simulink model "xPC_parker"  (Simulink 8.5)
settings: Solver=FixedStepDiscrete  StartTime=0.0  StopTime=inf  FixedStep=dts  RelTol=1e-3
InitFcn:
  | PARKER_DEPENDENCY
  | Parker_Multi_Axis_Init
  | Parker_ATI_Init
  | Parker_Home_Init
  | Parker_Davinci_Init
  | Parker_UDP_Init
  | Parker_LinIntPathPlan_Init
  | Parker_ScopeFormat_Init
  | Parker_magnetic_init
undefined symbols (not defined in the file): A, accel_filter_coeffs, ATI_torque_Nmm, B, counter_offset, DavinciFilterDen, DavinciFilterNum, DesiredPath, dt, dt_ENC, dt_trakstar, dts, dtudp, ENC_obs_filter_coeffs, encoder_counts, F, f_mag_desired_shape, filter_coeffs_bias, force_bias, forceDeadZone, FT_unbias_time, grav_vector, Home_in_TKbase, HOMING_dx, HOMING_num_joint, HOMING_tspan, HOMING_Vmov, inv_T, JOINT_Limits_Negative, JOINT_Limits_Postive, Kd, Ki_force, Kp, Kp_force, Kv_force, Low, N_acceleration, N_bias, N_ENC_obs_filter, N_obs_velocity, N_trakstar, N_velocity, Omega7IsLeftHanded, omni_scaling, PathPlanSpeed, pitch, quadrature_mode, R_FT2robot, R_omni, R_robot2TKbase, ResRateEpsilon, ResRateVelLimits, ResRateVelRatios, SafetyMargin, screw_pitch, torque_constant, trakstar_filter_coeffs, UDP_EN_Data2CMU, UDP_EN_DynAna, UDP_EN_VFRec ... (+6)
libraries: slrtlib x25, simulink x24, dspswit3 x15, xpcobsoletelib x15, xpcrtudplib x14, powerlib_meascontrol x3, xpcmeasurementcomputinglib x3, xpcconteclib x3
(part 3 of 3)

== system xPC_parker/Trajectory Planner/Task Input/UDP Visualize Superim ==
  x_ctr : Inport
  superim_cmd : Inport  Port=2
  Enable : EnablePort
  Demux1 : Demux  Outputs=7
  Mux3 : Mux  Inputs=3
  Pack : xpcobsoletelib/Utilities/Pack   datatypes={'double' 'double' 'double' 'double' 'double' 'double' 'double'}  byteAlign=1
  Parker_Send_to_VisualSuperim : xpcrtudplib/Legacy UDP/Send   ipAddress=255.255.255.255  ipPort=UDP_PORT_Send2VisualSuperim  localPort=-1  vblLen=off  sampletime=dtUDP_Data
  Rate Transition2 : RateTransition  OutPortSampleTime=dtUDP_Data
  STOP : Constant  Value=UDP_STOP
  wires:
  Pack/1 -> Parker_Send_to_VisualSuperim/1
  Mux3/1 -> Rate Transition2/1
  Rate Transition2/1 -> Demux1/1
  STOP/1 -> Mux3/3
  x_ctr/1 -> Mux3/1
  superim_cmd/1 -> Mux3/2
  Demux1/7 -> Pack/7
  Demux1/5 -> Pack/5
  Demux1/6 -> Pack/6
  Demux1/4 -> Pack/4
  Demux1/2 -> Pack/2
  Demux1/1 -> Pack/1
  Demux1/3 -> Pack/3

== system xPC_parker/Trajectory Planner/Task Input/position velocity acceleration ==
  velocity : Inport
  position : Inport  Port=2
  Desired Position : Subsystem
  Discrete Derivative1 : simulink/Discrete/Discrete Derivative  gainval=1.0  ICPrevScaledInput=[0;0;0]  InputProcessing=Inherited  OutMin=[]  OutMax=[]  OutDataType=fixdt(1, 16)  OutScaling=2^-10  DoSatur=off
  Mux : Mux  Inputs=3
  SatAcc : Saturate  UpperLimit=30  LowerLimit=-30
  PVA : Outport
  wires:
  Discrete Derivative1/1 -> SatAcc/1
  Mux/1 -> PVA/1
  SatAcc/1 -> Mux/3
  velocity/1 -> Desired Position/2(vel), Discrete Derivative1/1, Mux/2  "velocity"
  position/1 -> Desired Position/1(Pc)
  Desired Position/1(p_cmd) -> Mux/1

== system xPC_parker/Hybrid Motion PD Inverse Dynamics/Surf Norm Command/Conflict Check/Angle Compensation ==
  default_n : Inport
  surf_norm : Inport  Port=2
  Compensation : MATLAB Function  TreatAsAtomicUnit=on
  Constant : Constant  Value=12*pi/180
  Out1 : Outport
  wires:
  default_n/1 -> Compensation/2(N)
  surf_norm/1 -> Compensation/1(F)
  Constant/1 -> Compensation/3(angle_limit)
  Compensation/1(y) -> Out1/1

== system xPC_parker/Parker 404XR/Magnetic Tracker 125 Hz/process trak1/Filter1 ==
  in : Inport
  Discrete FIR Filter : DiscreteFir  CoefSource=Input port  SampleTime=dt_trakstar  AccumDataTypeStr=Inherit: Same as product output
  Gain : Gain  Gain=1/N_trakstar  SampleTime=dt_trakstar
  trakstar_filter_coeffs : Constant  Value=trakstar_filter_coeffs  SampleTime=dt_trakstar
  out : Outport
  wires:
  Gain/1 -> out/1
  in/1 -> Discrete FIR Filter/1
  Discrete FIR Filter/1 -> Gain/1
  trakstar_filter_coeffs/1 -> Discrete FIR Filter/2

== system xPC_parker/Parker 404XR/Magnetic Tracker 125 Hz/process trak2/Filter1 ==
  in : Inport
  Discrete FIR Filter : DiscreteFir  CoefSource=Input port  SampleTime=dt_trakstar  AccumDataTypeStr=Inherit: Same as product output
  Gain : Gain  Gain=1/N_trakstar  SampleTime=dt_trakstar
  trakstar_filter_coeffs : Constant  Value=trakstar_filter_coeffs  SampleTime=dt_trakstar
  out : Outport
  wires:
  trakstar_filter_coeffs/1 -> Discrete FIR Filter/2
  Discrete FIR Filter/1 -> Gain/1
  in/1 -> Discrete FIR Filter/1
  Gain/1 -> out/1

== system xPC_parker/Parker 404XR/Magnetic Tracker 125 Hz/process trak3/Filter1 ==
  in : Inport
  Discrete FIR Filter : DiscreteFir  CoefSource=Input port  SampleTime=dt_trakstar  AccumDataTypeStr=Inherit: Same as product output
  Gain : Gain  Gain=1/N_trakstar  SampleTime=dt_trakstar
  trakstar_filter_coeffs : Constant  Value=trakstar_filter_coeffs  SampleTime=dt_trakstar
  out : Outport
  wires:
  Gain/1 -> out/1
  in/1 -> Discrete FIR Filter/1
  Discrete FIR Filter/1 -> Gain/1
  trakstar_filter_coeffs/1 -> Discrete FIR Filter/2

== system xPC_parker/Parker 404XR/Magnetic Tracker 125 Hz/process trak4/Filter1 ==
  in : Inport
  Discrete FIR Filter : DiscreteFir  CoefSource=Input port  SampleTime=dt_trakstar  AccumDataTypeStr=Inherit: Same as product output
  Gain : Gain  Gain=1/N_trakstar  SampleTime=dt_trakstar
  trakstar_filter_coeffs : Constant  Value=trakstar_filter_coeffs  SampleTime=dt_trakstar
  out : Outport
  wires:
  trakstar_filter_coeffs/1 -> Discrete FIR Filter/2
  Discrete FIR Filter/1 -> Gain/1
  in/1 -> Discrete FIR Filter/1
  Gain/1 -> out/1

== system xPC_parker/Trajectory Planner/DaVinci MTM port: 2/DaVinci MTM/MTM Filter ==
  current_position : Inport
  Discrete FIR Filter : DiscreteFir  CoefSource=Input port  AccumDataTypeStr=Inherit: Same as product output
  Gain : Gain  Gain=1/20
  vel_filter_coeffs : Constant  Value=ones(20,1)
  vel_out : Outport
  wires:
  current_position/1 -> Discrete FIR Filter/1
  Gain/1 -> vel_out/1
  vel_filter_coeffs/1 -> Discrete FIR Filter/2
  Discrete FIR Filter/1 -> Gain/1

== system xPC_parker/Trajectory Planner/DaVinci MTM port: 2/UDP_feedback_to_MTM/Force Filter for MTM ==
  V_in : Inport  SampleTime=dts
  Discrete FIR Filter : DiscreteFir  CoefSource=Input port  SampleTime=dts  AccumDataTypeStr=Inherit: Same as product output
  Gain : Gain  Gain=1/100  SampleTime=dts
  filter_coeffs : Constant  Value=ones(100,1)  SampleTime=dt
  V_Out : Outport  SampleTime=dts
  wires:
  Gain/1 -> V_Out/1
  filter_coeffs/1 -> Discrete FIR Filter/2
  Discrete FIR Filter/1 -> Gain/1
  V_in/1 -> Discrete FIR Filter/1

== system xPC_parker/Trajectory Planner/Omega7/Feedback_to_omega7/force feedback filter ==
  V_in : Inport  SampleTime=dts
  Discrete FIR Filter : DiscreteFir  CoefSource=Input port  SampleTime=dts  AccumDataTypeStr=Inherit: Same as product output
  Gain : Gain  Gain=1/20  SampleTime=dts
  force feedback filter coef : Constant  Value=ones(20,1)  SampleTime=dts
  V_Out : Outport  SampleTime=dts
  wires:
  V_in/1 -> Discrete FIR Filter/1
  Discrete FIR Filter/1 -> Gain/1
  force feedback filter coef/1 -> Discrete FIR Filter/2
  Gain/1 -> V_Out/1

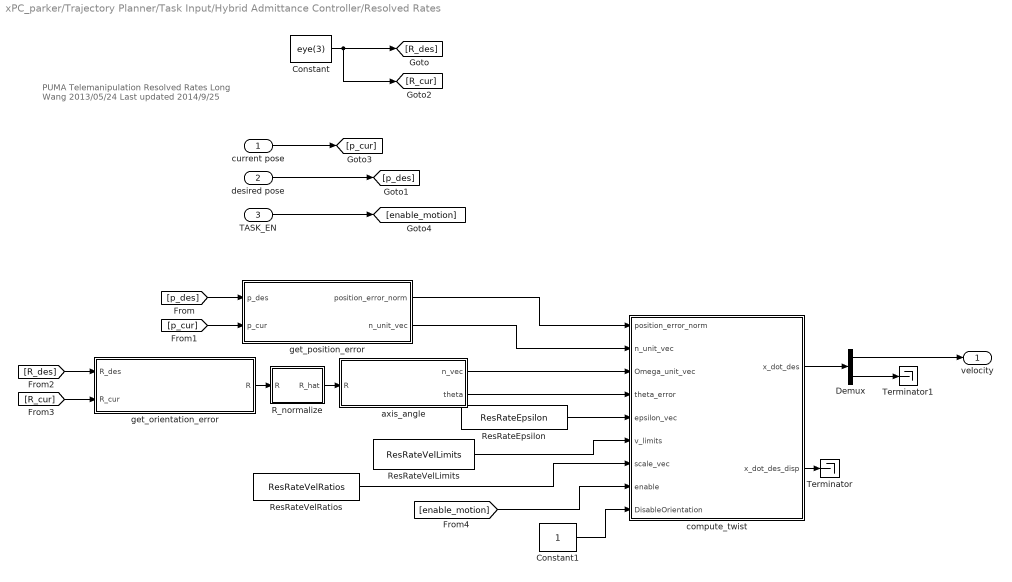
== system xPC_parker/Trajectory Planner/Task Input/Hybrid Admittance Controller/Resolved Rates ==
  note: PUMA Telemanipulation Resolved Rates
      | Long Wang
      | 2013/05/24
      | Last updated 2014/9/25
  current pose : Inport
  desired pose : Inport  Port=2
  TASK_EN : Inport  Port=3
  Constant : Constant  Value=eye(3)
  Constant1 : Constant
  Demux : Demux  Outputs=2
  R_normalize : MATLAB Function  TreatAsAtomicUnit=on
  ResRateEpsilon : Constant  Value=ResRateEpsilon
  ResRateVelLimits : Constant  Value=ResRateVelLimits
  ResRateVelRatios : Constant  Value=ResRateVelRatios
  Terminator : Terminator
  Terminator1 : Terminator
  axis_angle : MATLAB Function  TreatAsAtomicUnit=on
  compute_twist : MATLAB Function  TreatAsAtomicUnit=on
  get_orientation_error : MATLAB Function  TreatAsAtomicUnit=on
  get_position_error : MATLAB Function  TreatAsAtomicUnit=on
  velocity : Outport
  wires:
  get_position_error/1(position_error_norm) -> compute_twist/1(position_error_norm)
  get_position_error/2(n_unit_vec) -> compute_twist/2(n_unit_vec)
  ResRateVelLimits/1 -> compute_twist/6(v_limits)
  ResRateEpsilon/1 -> compute_twist/5(epsilon_vec)
  desired pose/1 -> [p_des]
  Constant/1 -> [R_cur], [R_des]
  current pose/1 -> [p_cur]
  ResRateVelRatios/1 -> compute_twist/7(scale_vec)
  get_orientation_error/1(R) -> R_normalize/1(R)
  TASK_EN/1 -> [enable_motion]
  [p_des] -> get_position_error/1(p_des)
  [p_cur] -> get_position_error/2(p_cur)
  [R_des] -> get_orientation_error/1(R_des)
  [R_cur] -> get_orientation_error/2(R_cur)
  [enable_motion] -> compute_twist/8(enable)
  axis_angle/1(n_vec) -> compute_twist/3(Omega_unit_vec)
  axis_angle/2(theta) -> compute_twist/4(theta_error)
  R_normalize/1(R_hat) -> axis_angle/1(R)
  compute_twist/2(x_dot_des_disp) -> Terminator/1
  Constant1/1 -> compute_twist/9(DisableOrientation)
  compute_twist/1(x_dot_des) -> Demux/1
  Demux/1 -> velocity/1
  Demux/2 -> Terminator1/1

== system xPC_parker/Trajectory Planner/Task Input/Superimposed Motion/Motion Projector1 ==
  n : Inport
  Fm : Inport  Port=2
  Projector : MATLAB Function  TreatAsAtomicUnit=on
  v_allowed : Outport
  wires:
  n/1 -> Projector/2(N)
  Projector/1(y) -> v_allowed/1
  Fm/1 -> Projector/1(F)

== system xPC_parker/Trajectory Planner/Task Input/Superimposed Motion/Velocity Filter ==
  current_position : Inport
  Discrete FIR Filter : DiscreteFir  CoefSource=Input port  AccumDataTypeStr=Inherit: Same as product output
  Gain : Gain  Gain=1/N_velocity
  vel_filter_coeffs : Constant  Value=vel_filter_coeffs
  vel_out : Outport
  wires:
  current_position/1 -> Discrete FIR Filter/1
  Gain/1 -> vel_out/1
  vel_filter_coeffs/1 -> Discrete FIR Filter/2
  Discrete FIR Filter/1 -> Gain/1

== system xPC_parker/Trajectory Planner/Task Input/position velocity acceleration/Desired Position ==
  note: This gain is helping to
      | magnify the error,
      | as a "spring"
  Pc : Inport
  vel : Inport  Port=2
  Gain : Gain  Gain=dt
  Gain1 : Gain  Gain=10
  MATLAB Function : MATLAB Function  TreatAsAtomicUnit=on
  N-Sample Switch : dspswit3/N-Sample Switch  N=1  reset=off  TriggerType=Rising edge  Ts=dt
  SatPos : Saturate  UpperLimit=JOINT_Limits_Postive  LowerLimit=JOINT_Limits_Negative
  Sum1 : Sum  Inputs=|++
  Switch : Switch  Criteria=u2 > Threshold
  Unit Delay : UnitDelay  InitialCondition=zeros(3,1)  SampleTime=-1
  p_cmd : Outport
  wires:
  Gain/1 -> Gain1/1  "dx"
  SatPos/1 -> p_cmd/1
  vel/1 -> Gain/1
  Switch/1 -> Unit Delay/1, SatPos/1
  Sum1/1 -> Switch/1
  MATLAB Function/1(y) -> Switch/2
  Pc/1 -> [pc]
  [pc] -> Sum1/1
  N-Sample Switch/1 -> Switch/3
  Unit Delay/1 -> N-Sample Switch/2
  [pc] -> N-Sample Switch/1
  Gain1/1 -> Sum1/2, MATLAB Function/1(u)

== matlab function Trajectory Planner/Omega7/Omni Task Ref/Task Reference ==
  data: b_R_o input double; scaling input double; x_cmd output double; enPos input double; enOri input double; vlim input double; dt input double; x_tele input double; x_prev input double; x_s output double; x_s_prev input double
function [x_cmd, x_s ] = taskReference(b_R_o,scaling, enPos,enOri,vlim,dt,x_tele,x_prev,x_s_prev)
%#codegen
% ################################################################################################
% NOTES:
% need to implement orientation and spatial teleoperation
%
% ################################################################################################

% TELEOPERATION

if (enOri==1) % spatial control overrides position control --------------------------------
    x_s=x_tele;     % start position redefined
    dx=[0;0;0]; % assume motion is zero (safety)
    x_cmd=x_prev+dx; % increment commanded position by displacement
elseif (enPos==1) % if spatial control note desired, check for position control -----------
    x_s=x_tele;     % start position redefined
    dx=b_R_o*scaling(1)*(x_tele-x_s_prev); % scale displacement and rotate to robot frame
    M=norm(dx);
    xlim=vlim*dt; % unit in mm/sec
    if M>xlim
        alpha=xlim/M;
    else
        alpha=1;
    end
    x_cmd=x_prev+alpha*dx; % increment commanded position by displacement
else        % do nothing and hold previous position ---------------------------------------
    x_cmd=x_prev;
    x_s=x_tele;
end

== matlab function Trajectory Planner/Task Input/Motion Projector/Projector ==
  data: F input double; N input double; y output double
function y = fcn(F,N)

Omega_f = N * N';
Omega_m = eye(3) - Omega_f;

y = Omega_m * F;

== matlab function Force Sensor/Contact_Estimation/Ball Contact Correction ==
  data: error_mag output double; Contact output double; wrench input double; tip_offset input double; r_ball input double; f_in_b output double; dx_in_b output double; R_f2b input double; surf_norm output double; F_thres input double; LowForce_thres input double; M_thres input double; surf_norm_prev input double; LowForceContact output double; LowForceSeparate output double
function [error_mag,Contact,f_in_b,dx_in_b,surf_norm,LowForceContact,LowForceSeparate]=fcn(wrench,tip_offset,r_ball,R_f2b,F_thres,LowForce_thres,M_thres,surf_norm_prev)
%#codegen
%% By Long Wang, 2014/8/8
%   this func will
%   1) correct the contact tip position based on the
%   2) compute the estimate error between force measurement and moment
%   measurement
%% variables:
%   tip_offset [mm] is the vector of the tip in force sensor frame
%   r_ball [mm] is the radius of the ball sephear
%   wrench [N,Nmm]is the wrench measured in force sensor frame
%   R_f2b is the rotation matrix from force sensor frame to robot base
%   f [N] is the measured force
%   dx [mm] is the contact tip position in force sensor frame
%   error_mag [Nmm] is the moment error magnitude between force measurement and moment
wrench = wrench(:);
f = wrench(1:3);
m = wrench(4:6);
epsilon_f = F_thres;

if norm(f)<epsilon_f % if it is just noise
    error_mag = 0;
    n_hat_in_f = zeros(3,1);
else
    n_hat_in_f = f/norm(f);
    dx = -n_hat_in_f*r_ball;
    error = cross((tip_offset+dx),f)-m;
    error_mag = norm(error);
end
epsilon_m = M_thres; %error in moment equation in Nmm

if error_mag<epsilon_m
    %%  compute the contact point location
    f_in_b = R_f2b*f;
    surf_norm = R_f2b*n_hat_in_f;
    %     dx_in_b = R_f2b*dx;
    dx_in_b = -r_ball*surf_norm_prev; % use the previous norm direction to update, this will smooth everything but still keep contact detection responsive
    %%  confirm contact is above certain threshold
    contact_thresh = F_thres;
    if norm(f_in_b)>contact_thresh
        Contact = 1;
    else
        Contact = 0;
        surf_norm = zeros(3,1);
    end
    %%  detect low force contact flag
    if norm(f_in_b)>LowForce_thres
        LowForceContact = 1;
        LowForceSeparate = 0;
    else
        LowForceContact = 0;
        LowForceSeparate = 1;        
    end
else
    f_in_b = zeros(3,1);
    dx_in_b = zeros(3,1);
    Contact = 0;
    surf_norm = zeros(3,1);
    LowForceContact = 0;
    LowForceSeparate = 1;
end

== matlab function Trajectory Planner/Homing/Homing Procedure ==
  data: dt input double; tspan input double; V_mov input double; home_pos input double; switches input double; q_prev input double; q_des output double; qd_des output double; qdd_des output double; ready output double; stop_flag input double; A_in input double; prev_status input double; A_out output double; cur_status output double; reset output double; q_cur input double; lsf_in input double; lsf_out output double
% this function executes a homing sequence for the parallel robots
% status definition:
%       1: keep homing
%       0: stop homing
% stop flag definition:
%       0: all limit switches have not been reached
%       1: limit switches reached, calculate trajectory to home config
%       2: run 5th order poly
%       3: home complete - reset and hold position
%       4: turn off reset, hold at 0

function [q_des,qd_des,qdd_des,ready,A_out,cur_status,reset,lsf_out] = homing(dt,tspan,V_mov,home_pos,switches,q_prev,stop_flag,A_in,prev_status,q_cur,lsf_in)
% V_mov=5; % leg velocity while homing (mm/s)
% tspan=10;    % time to execute path plan (sec)
N=length(q_prev);
qd_des=zeros(N,1); % default desired velocity
qdd_des=zeros(N,1); %default desired acceleration

% read limit switches
% when limit switches are reached, switch=1
status=ones(N,1)-switches;    % update triggered switches
lsf_out=lsf_in.*status;
if stop_flag==1
    dx=home_pos;    % total displacement
    A_out=zeros(N,4);   % allocate memory for coefficients

    % construct coefficients
    for i=1:N
        A_out(i,:)=[q_prev(i),10*dx(i), -15*dx(i), 6*dx(i)];
    end
    cur_status=1;
    cur_t=cur_status*dt/tspan;
    T=[1;cur_t^3;cur_t^4;cur_t^5];    % exponential time vector
    q_des=A_out*T;  % current desired position 
    ready=2;        % continue with path plan (should be 2)
    reset=0;
elseif stop_flag==2
    
    if prev_status>=(tspan/dt)    % reached position goal
        T=[1;1;1;1];
        q_des=A_in*T;
        cur_status=prev_status;
        A_out=[q_des,zeros(N,3)];
        ready=3;
        reset=0;
    else    % continue on the trajectory
        cur_t=prev_status*dt/tspan; % current normalized time [0 -> 1]
        T=[1;cur_t^3;cur_t^4;cur_t^5];    % exponential time vector
        q_des=A_in*T;  % current desired position
        cur_status=prev_status+1; % update status step
        A_out=A_in; % maintain current coefficients  
        ready=2;
        reset=0;
    end
elseif stop_flag==3
    cur_status=0;
    A_out=zeros(N,4);
    q_des=q_cur;
    ready=4;
    reset=1;
elseif stop_flag==4
    cur_status=0;
    A_out=zeros(N,4);
    q_des=q_cur*0;
    ready=4;
    reset=0;
else
    % check homing status    
    if (sum(lsf_out))==0   % all limit switches have been reached
        q_des=q_prev;       % stop motion
        ready=1;            % homing finished
        cur_status=0;
        A_out=zeros(N,4);
        reset=0;
    else    % continue homing
        q_des=q_prev + status.*V_mov*dt;   % move legs that have not reached goal
        ready=0;            % homing not finished
        cur_status=0;
        A_out=zeros(N,4);
        reset=0;
    end
end

== matlab function Trajectory Planner/Omega7/Feedback_to_omega7/Force Filter ==
  data: f input double; f_delta input double; R_m2s input double; f_out output double; f_prev input double; f_out_in_master output double
function [f_out,f_out_in_master] = forceFilter(f,f_delta,R_m2s,f_prev)
%#codegen
f_error = f-f_prev; % current gap in input/output force
% fdelta=0.002; % max change of force per time step
f_out=zeros(4,1);
for i=1:3
    if abs(f_error(i))>f_delta
        f_out(i) = f_prev(i)+sign(f_error(i))*f_delta;
    else
        f_out(i) = f(i);
    end
end
f_out(4)=f(4); % gripper force is not filtered
%%  rewrite in master frame
R_s2m = R_m2s';
f_out_in_master = zeros(4,1);
f_out_in_master(1:3) = R_s2m*f_out(1:3);
f_out_in_master(4) = f(4);

== matlab function Trajectory Planner/DaVinci MTM port: 2/Davinci Task Ref/Task Reference ==
  data: MSG_TYPE input double; x_cmd output double; x_des input double; R_des input double; xs input double; R_cmd output double; Rs input double; Task_EN output double
function [x_cmd,R_cmd,Task_EN] = fcn(MSG_TYPE,x_des,R_des,xs,Rs)
%#codegen
% x_cmd -> position command reference
% R_cmd -> orientation command reference written using quaternion (fake/virtual if Parker XYZ does not have a wrist)
Task_EN = bitand(uint8(floor(MSG_TYPE)),1);
if Task_EN ==1
    x_cmd = x_des;
    R_cmd = R_des;
else
    x_cmd = xs;
    R_cmd = Rs;
end

== matlab function Hybrid Motion PD Inverse Dynamics/Motion Projector/Projector ==
  data: F input double; N input double; y output double
function y = fcn(F,N)

Omega_f = N * N';
Omega_m = eye(3) - Omega_f;

y = Omega_m * F;

== matlab function Hybrid Motion PD Inverse Dynamics/Force Projector 1/Projector ==
  data: F input double; N input double; y output double
function y = fcn(F,N)

Omega_f = N * N';

y = Omega_f * F;

== matlab function Hybrid Motion PD Inverse Dynamics/Force Projector 2/Projector ==
  data: F input double; N input double; y output double
function y = fcn(F,N)

Omega_f = N * N';

y = Omega_f * F;

== matlab function Force Sensor/Convert from Voltage to Wrench ==
  data: V input double; W output double; A input double; inv_T input double
function W = Convert_Function(V,A,inv_T)%A_vec,p)

W = inv_T*A*V;

== matlab function Hybrid Motion PD Inverse Dynamics/normalize ==
  data: u input double; y output double
function y  = fcn(u)
%#codegen
mag = norm(u);
if mag>0
    y = u/mag;
else
    y = [0;0;0];
end

== matlab function Trajectory Planner/Task Enable Logic/MATLAB Function ==
  data: MSG_TYPE input double; Task_EN output double
function Task_EN = fcn(MSG_TYPE)
%#codegen
Task_EN = bitand(uint8(floor(MSG_TYPE)),1);

== matlab function Trajectory Planner/Quintic Polynomial/trigger detection/MATLAB Function ==
  data: trig input double; enable output double; trig_history input double
function enable= fcn(trig,trig_history)
%#codegen
%%  This func is just to detect a rising trigger
%   Once this rising trigger detected, this manual enable will be locked
%   until mode change
if trig_history==0
    if trig==0
        enable=0;
    else
        enable=1;
    end
else
    enable = 1;
end

== matlab function Trajectory Planner/Task Input/position velocity acceleration/Desired Position/MATLAB Function ==
  data: u input double; y output double
function y = get_norm(u)
%#codegen

y = norm(u,2);

== matlab function Trajectory Planner/Path Following/Path Planning ==
  data: dState input double; x output double; cState input double; path input double; vel input double; dt input double; dt_prev input double; x_cur input double; state output double; dt_cur output double; distance output double; pauseFLAG input double; sLimit input double; READY_TIME input double
function [x, state, dt_cur, distance] = InsertionPlan(dState,cState,path,vel,dt,dt_prev,x_cur,pauseFLAG,sLimit,READY_TIME)
%#codegen
% This is for single axis insertion system
% The variable 'dstate' selects what part of the insertion process the robot is currently in (cState):
% 1 -> moving toward starting position
% 2 -> ready to execute
% 3 -> running
% 4 -> finished

%  Format of path
% path(1,:) => path s point
% path(2,:) => x
% path(3,:) => y
% path(4,:) => z

% the 'pauseFLAG' is set to 1 if the user wishes to pause current progress,
% in effect the dt is set to 0

% 'sLimit' sets the maximum displacement along the path (parameterized by
% distance 's').  A positive value enforces a limit to that point, a 
% negative value sets no limitation.

% Set state for this time step
if dState>cState
    tState=cState;
else
    tState=dState;
end


switch tState
    case 1; % Move to initial position
        x=path(2:4,1);
        if norm(x-x_cur)<0.001
            state=2;
        else
            if norm(x-x_cur)>2
                v = vel;
            else 
                v = 1;
            end
            state=1;
            n = (x-x_cur)/norm(x-x_cur);
            x = x_cur + v*dt*n;
        end
        dt_cur=0;
        distance=0;
    case 2 % Holding at initial insertion pose
        x=x_cur;
        dt_cur=dt_prev+dt;
        state=2;
        distance=0;
        if dt_prev>READY_TIME % wait READY_TIME seconds before moving to path follow phase
            dt_cur=0;
            state=3;
        end
    case 3 % start interpolation
        
        distance=vel*dt_prev;
        
        if (sLimit>0)
            if distance>sLimit
                pauseFLAG=1; % overwrite pauseFLAG so that dt_cur doesn't increase     
            end
        end
        
        if distance > path(1,end)
            distance=path(1,end);   % hold at end of path
            x=path(2:4,end);
            state=4;
        else
            state=3;
           x=[interp1(path(1,:),path(2,:),distance);
              interp1(path(1,:),path(3,:),distance);
              interp1(path(1,:),path(4,:),distance)];
 
        end
        if (pauseFLAG==1)
            dt_cur=dt_prev; % hold time step
        else
            dt_cur=dt_prev+dt; % update time step
        end
        
        
    otherwise
        x=x_cur;
        dt_cur=0;
        state=4;
        distance=0;
end

== matlab function Trajectory Planner/Path Following/Scan Pattern Filter ==
  data: x_des input double; x_cmd output double; cState input double; xc input double
function x_cmd = fcn(x_des,cState,xc)
%#codegen
x_cmd = zeros(3,1);
x_cmd = x_des;
if cState==3
    x_cmd(3) = xc(3);
end

== matlab function Hybrid Motion PD Inverse Dynamics/Force Projector 3/Projector ==
  data: F input double; N input double; y output double
function y = fcn(F,N)

Omega_f = N * N';

y = Omega_f * F;

== matlab function Hybrid Motion PD Inverse Dynamics/Surf Norm Command/Conflict Check/Angle Compensation/Compensation ==
  data: F input double; N input double; y output double; angle_limit input double
function y = fcn(F,N,angle_limit)
%% angle_limit [rad], to specify the compensation angle to lift up the projection out of the plane
dot_prod = F'*N;

if dot_prod<sin(angle_limit)
    Omega_f = N * N';
    Omega_m = eye(3) - Omega_f;
    projection = Omega_m * F;
    L_projection = norm(projection);
    y = projection + N*tan(angle_limit)*L_projection;
    y = y/norm(y);
else
    y = F;
end

== matlab function Trajectory Planner/Task Input/Hybrid Admittance Controller/Resolved Rates/R_normalize ==
  data: R input double; R_hat output double
function R_hat = R_norm(R)
%#codegen
rx = R(:,1);
rx = rx/norm(rx);
ry = R(:,2);
ry = ry/norm(ry);
rz = cross(rx,ry);
rz = rz/norm(rz);
R_hat = [rx,ry,rz];
end

== matlab function Trajectory Planner/Task Input/Hybrid Admittance Controller/Resolved Rates/axis_angle ==
  data: R input double; n_vec output double; theta output double
function [n_vec, theta] = get_axis_angle(R)
%#codegen
% Jason Pile
%axis_angle(R) gives the rotation axis and the rotation angle extracted
%from rotation matrix R
%   n_vec=unit vector along rotation axis
%   theta=rotation angle about rotation axis
    theta=acos(1/2*(trace(R)-1));
    if abs(theta)<(10^-4)
        n_vec=[1;0;0];
    elseif abs(theta-pi)<(10^-4)
        n_vec=[-1;0;0];        
    else
        n_cross=1/(2*sin(theta))*(R-R');
        n_vec=[-n_cross(2,3);n_cross(1,3);-n_cross(1,2)];
        n_vec=n_vec/norm(n_vec);
    end
end

== matlab function Trajectory Planner/Task Input/Hybrid Admittance Controller/Resolved Rates/get_orientation_error ==
  data: R_des input double; R_cur input double; R output double
%#codegen
function R  = GetOrientationErr(R_des,R_cur)
% Long Wang
% 2013/06/02
% orientation error R_des=R*R_cur is a rotayionn sequence in world frame
R = R_des * (R_cur');

== matlab function Trajectory Planner/Quintic Polynomial/5th Order Polynomial/Embedded MATLAB Function ==
  data: p output double; p_des input double; p_curr input double; tf input double; tc input double; pdot output double; pdotdot output double; conf input double; confn output double; t0 input double; t0n output double; p0n output double; p0 input double; enable input double; RECORD output double
function [p,pdot,pdotdot,confn,t0n,p0n,RECORD] = fifth_order_p(p_des,p_curr,tf,tc,conf,t0,p0,enable)

n = 3;
RECORD = 0;

if enable == 0                  % Configuration space is not used (pdot = 0). 
    p = p_curr;
    pdotdot = zeros(n,1);
    pdot = zeros(n,1);          % However we do want to record the current 
    confn = 0;                  % position in order to be ready as soon 
    t0n = tc;                   % as the enable becomes 1. 
    p0n = p_curr;
else
    if (p_des-p0)'*(p_des-p0) > 0
        if conf == 0                % conf = 0 means that the 5th order poly 
            p0n = p0;               % is not configured for the desired trajectory.
            t0n = tc;               % Therefore, the block is initialized.
            confn = 1;
            pdot = zeros(n,1);
            p = p0;
            pdotdot = zeros(n,1);
        else
            p0n = p0;
            t0n = t0;
            confn = conf;
            % 5th order polynomial
            a0 = p0;
            a4 = -15*(p_des-p0);
            a3 = -2/3 * a4;
            a5 = -2/5 * a4;
            t = tc-t0;
            tau = t/tf;
            if t < tf
                RECORD = 1;
                p = a0 + a3 * tau^3 + a4 * tau^4 + a5 * tau^5;
                pdot = 3*a3*t^2/tf^3 + 4*a4*t^3/tf^4 + 5*a5*t^4/tf^5;
                pdotdot = 6*a3*t/tf^3 + 12*a4*t^2/tf^4 + 20*a5*t^3/tf^5;
            else
                p = p_des;
                pdot = zeros(n,1);
                pdotdot = zeros(n,1);
                p0n = p_des;
            end
        end
    else
        p = p_des;
        pdot = zeros(n,1);
        pdotdot = zeros(n,1);
        confn = 0;
        p0n = p0;
        t0n = t0;
    end
end
%------------------------------------------------------------------------

== matlab function Trajectory Planner/Task Input/Hybrid Admittance Controller/Resolved Rates/get_position_error ==
  data: p_des input double; p_cur input double; position_error_norm output double; n_unit_vec output double
%#codegen
function [position_error_norm,n_unit_vec] = GetPositionErr(p_des,p_cur)
% Long Wang 2013/06/02
p_des = p_des(:); % make sure column vector
p_cur = p_cur(:);
position_error_vec = p_des-p_cur;
position_error_norm = norm(position_error_vec);
%% compute linear velocity direction
if position_error_norm==0
    n_unit_vec = [1;0;0];
else
    n_unit_vec = position_error_vec/position_error_norm;
end

== matlab function Trajectory Planner/Task Input/Superimposed Motion/MATLAB Function1 ==
  data: R input double; n output double; theta output double
function [n,theta] = fcn(R)
%#codegen

[n,theta] = AxisAngle(R);

== matlab function Trajectory Planner/Task Input/Superimposed Motion/Cycloid Motion ==
  data: x_des output double; x_ctr output double; Task_EN input double; dt input double; SetCycloidPro input double; Vmax input double; CtrVelocity input double; SetRotation input double; xdes_prev input double; x_ctr_prev input double; phi input double; CycloidProPrev input double; phiNext output double; CycloidProNext output double
function [x_des,x_ctr,phiNext,CycloidProNext]    =CycloidMotionControl(Task_EN, dt,SetCycloidPro,Vmax,CtrVelocity,SetRotation,xdes_prev,x_ctr_prev,phi,CycloidProPrev)
%#codegen
%%  Long Wang, 2014/11/3
%%  Cycloid motion V2.0
%   Task_EN -> Task enable
%   EN=0 => Disabled
%           Ready to take new cycloid motion profile parameter, 
%           note that the only two parameters are: eta, b; see Nabil and Long's notes
%   EN=1 => In the process of a superimposed telemanipulation (the coag button being pressed)
%   SetCycloidPro, CycloidProPre description:
%   vec = [eta,b]
%       eta,b are coefficients for motion equations:
%           x = eta*b phi - b sin(phi)
%           y = eta*b - b cos(phi)
%       Note that here, we want prolate cycloid, so eta->(0,1)
%   CtrVelocity -> set the desired velocity of the center of the "roller" for the current execution.
%   phi, phiNext -> the angle variable which drives the motion equations
%   Vmax    ->  the maxium velocity of the parker in superimposed motion
%               mode
%   v_ctr is the velocity of center 
%   vel_XY    ->  2D velocity in cycloid motion local frame
%   vel_des   ->  3D velocity relative to cycloid motion local origin, written in robot base frame.
%   Rotation, pRotation, SetRotation  ->    Rotation Matrix R_local2world, defined by
%                                           the velocity command given by user.
%                                           Rotation is the one currently
%                                           used; pRotation is the one from
%                                           previous time step; SetRotation
%                                           is the desired one.
CycloidProNext = SetCycloidPro;
if Task_EN
    eta = CycloidProPrev(1);
    b = CycloidProPrev(2);
%     output_args = GetCycloidMotion('CtrVel',[eta,b],[phi,CtrVelocity]);
%     phidot = output_args(1);
%     vel_XY = output_args(2:3);
%       limit the velocity on the trajectory: 
%       if the norm of computed vel_XY is larger Vmax, then use Vmax to
%       compute the velocity on the cycloid trajectory and also for phidot
%     if norm(vel_XY)>Vmax
     if CtrVelocity==0
        Vmax = 0;    
        phi = pi;
     end
        output_args = GetCycloidMotion('PtVel',[eta,b],[phi,Vmax]);
        phidot = output_args(1);
        vel_XY = output_args(2:3);
        CtrVelocity = eta*b*phidot;
%     end
    phiNext = phi + phidot*dt;
    vel_des = SetRotation*[vel_XY;0];
    x_des = xdes_prev + vel_des*dt;
    CycloidProNext = CycloidProPrev;
    % the following is just for debugging
    x_ctr = x_ctr_prev + SetRotation*[CtrVelocity;0;0]*dt;
else
    phiNext = pi;
    CycloidProNext = SetCycloidPro;
    x_des = xdes_prev;
    % the following is just for debugging
    x_ctr = xdes_prev;
end

== matlab function Trajectory Planner/Task Input/Superimposed Motion/normalize1 ==
  data: v_ctr output double; n input double; R output double; vel input double; eps input double; R_prev input double
function [v_ctr,R]  = GetRotation(n,vel,eps,R_prev)
%#codegen
%%  Long Wang, 2014/11/3
%   This func will determine the plane and frame that the cycloid motion
%   defined
%   Case 1: 
%       If n is an arbitrary vector, it means that the robot has been
%       commanded to servo force along n direction and servo motion in n
%       perpendicular plane
%   Case 2:
%       If n is all zeors, it means that the robot has been commanded
%       freely to servo motion in 3D space, no constraint about the motion
%       space.
%       In this case then we want to do the cycloid in XY plaine.
%   Input:
%   n   ->  The force control direction, or the norm of the cycloid motion
%           plane
%   vel ->  Current velocity command from the user
%   eps ->  the deadzone for velocity
%   n_vel_prev, n_vel   ->  the direction velocity unit vector
% 
%%  Calculate n_vel
if norm(n)==0
    n = [0;0;1];
    Omega_f = n * n';
    Omega_m = eye(3) - Omega_f;
    vel = Omega_m * vel;
end
if norm(vel)>eps
    cycloid_enable = 1;    
else
    cycloid_enable = 0;   
end
 
if cycloid_enable==1 % if cycloid_enable, recalculate R, otherwise use the one before 
    %%  Calculate R
    n_vel = vel/norm(vel);
    Rz = n(:);    % both n, and n_vel are already normalized; n is normalized in other blocks.
    Rx = n_vel(:); % garuantee to be column vector
    Ry = cross(Rz,Rx);
    Ry = Ry/norm(Ry); % normalize R_y
    Rx = cross(Ry,Rz); % recalculate R_x to ensure Rx, Ry, Rz are althorganal
    R = [Rx, Ry, Rz];
    v_ctr = norm(vel);  % v_ctr is the velocity of the center of the "roller" along local x axis, note that it is always scalar and positive.
else
    R = R_prev;
    v_ctr = 0;
end

== matlab function Trajectory Planner/Task Input/Superimposed Motion/MATLAB Function ==
  data: R_des input double; omegaMax input double; dt input double; R_prev input double; R output double
function R = RotationSaturation(R_des,omegaMax,dt,R_prev)
%#codegen
%%  Long Wang, 2014/12/11, this function will limit the maxium rotation change
detR = R_des*R_prev';
[n,theta] = AxisAngle(detR);
if abs(theta)<(omegaMax*dt)
    R = R_des;
else
    thetaMax = sign(theta)*(omegaMax*dt);
    detR = RotationAxisAngle(n,thetaMax);
    R = detR*R_prev;
end

== matlab function Trajectory Planner/Task Input/Superimposed Motion/Motion Projector1/Projector ==
  data: F input double; N input double; y output double
function y = fcn(F,N)

Omega_f = N * N';
Omega_m = eye(3) - Omega_f;

y = Omega_m * F;

== matlab function Force Sensor/Force Stop/MATLAB Function ==
  data: u input double; y output double
function y = not(u)
%#codegen

y = 1-u;

== matlab function Parker 404XR/Magnetic Tracker 125 Hz/compute robot pose ==
  data: FT_X_sr input double; FT_Y_sr input double; probe_offset_in_FT input double; BallCenter_in_TK output double; R_FT2TKbase output double; fail output double
function [BallCenter_in_TK,R_FT2TKbase,fail] = fcn(FT_X_sr,FT_Y_sr,probe_offset_in_FT)
%#codegen
%%  By Long Wang, 2015/7/9
%   Inputs:
%       FT_X_sr -> sensor attached on force sensor holder, aligned with X+
%           of FT
%       FT_Y_sr -> sensor attached on force sensor holder, aligned with Y+
%           of FT
%       target1 -> sensor attached on the 1st target
%       target2 -> sensor attached on the 2nd target
%       probe_offset_in_FT  -> the vector pointing from the EM tracker
%           holder origin to the ball probe center, written in force sensor
%           Frame
%       R_robot2TKbase ->   the rotation matrix from robot base to tracker
%       base
%%  Design specs:
%
[BallCenter_in_TK,R_FT2TKbase,fail] = parkerGetFrame_TK2FT(...
                    FT_X_sr,FT_Y_sr,probe_offset_in_FT);

== matlab function Force Sensor/Contact_Estimation/Compute Contact in TK ==
  data: BallCenter_in_TK input double; TK_fail input double; c_in_robot input double; dx_in_robot input double; c_in_TK_tracked output double; R_robot2TK input double; Home_in_TK input double; c_in_TK_robkin output double
function [c_in_TK_tracked,c_in_TK_robkin] = compute_contact_in_TK(BallCenter_in_TK,TK_fail,c_in_robot,dx_in_robot,R_robot2TK,Home_in_TK)
%#codegen
%%  By Long Wang, 2015/7/10
%%   Inputs:
%       BallCenter_in_TK    ->      Current ball center measured by TK, in TK
%                                  frame
%       dx_in_robot     ->  the contact location offset w.r.t to ball
%                           center
%       c_in_robot      ->  the contact location written in robot base
%%  Outputs:
%     c_in_TK_tracked   ->  the contact point location calculated by the
%                           tracker sensed ball center + dx
%     c_in_TK_robkin    ->  the contact point location calculated by the
%                           robot kinematics with registered transformation
c_in_TK_tracked = BallCenter_in_TK + R_robot2TK*dx_in_robot;
c_in_TK_robkin = Home_in_TK + R_robot2TK*c_in_robot;

== matlab function Trajectory Planner/safety check/false detection ==
  data: pva_cmd input double; pva_allowed output double; pva_prev input double; error_flag output double; error_prev input double
function [pva_allowed,error_flag] = fcn(pva_cmd,pva_prev,error_prev)
%#codegen
%%  This func is a safety check
%   once the system received some illegal command, the system will be
%   locked for diagnostic purpose
error_flag = 0;
if sum(isnan(pva_cmd))~=0
    error_flag = 1;
end
if sum(isinf(pva_cmd))~=0
    error_flag = 1;
end
if sum(abs(pva_cmd(1:3))>250)~=0 % out of stroke command
    error_flag=1;
end
if error_prev % once faulty, lock down.
    error_flag = 1;
end

if error_flag
    pva_allowed = pva_prev;
else
    pva_allowed = pva_cmd;
end

== matlab function Trajectory Planner/Omega7/MATLAB Function ==
  data: online input double; enable output double; GP input double; GP_thresh input double; LeftHand input double
function enable = fcn(online,GP,GP_thresh,LeftHand)
%#codegen
if online==1
    if LeftHand==1
        if GP>-GP_thresh
            enable = 1;
        else
            enable = 0;
        end
    else
        if GP<GP_thresh
            enable = 1;
        else
            enable = 0;
        end        
    end
else
    enable = 0;
end
end

== matlab function Trajectory Planner/Task Input/Hybrid Admittance Controller/Resolved Rates/compute_twist ==
  data: position_error_norm input double; n_unit_vec input double; Omega_unit_vec input double; theta_error input double; epsilon_vec input double; v_limits input double; scale_vec input double; x_dot_des output double; enable input double; x_dot_des_disp output double; DisableOrientation input double
%#codegen

function [x_dot_des,x_dot_des_disp ]= compute_twist(position_error_norm,n_unit_vec, Omega_unit_vec, theta_error,epsilon_vec,v_limits,scale_vec,enable,DisableOrientation)
%% compute_twist :
%   Description:    This embedded matlab function computes the desired twist
%                   of the end-effector to follow a straight line through p_curr
%                   and p_des and bring the R_curr to R_des using angle/axis
%                   representation
%
%   References:     Siciliano, Sciavicco, Villani, Oriolo, Robotics: Modelling, Planning and Control
%                   1. angle/axis pg 52
%                   2. trajectories pg 161
%
%                   Nabil's notes on Resolved Rate Algorithm
%
%   Inputs:         1. p_des is the desired end effector position
%                   2. R_des is the desired end effectror orientation
%                   3. p_curr is the current position of the robot's operational point
%                   5. R_curr is the current orientation of the robot's tool
%   Outputs:        1. x_des is the desired twist of the robot end-effector
%                   2. theta is the orientation error (to be removed in final version)
%--------------------------------------------------------------------------
if enable == 1  % if motion is enabled
    Vmin = v_limits(1,1); % [m/s]
    Vmax = v_limits(2,1); % [m/s]
    OmegaMin = v_limits(3,1);   %rad/s
    OmegaMax = v_limits(4,1);   %rad/s
    
    position_epsilon=epsilon_vec(1);
    orientation_epsilon=epsilon_vec(2);
    
    %%  check for convergence
    lin_vel_ratio = scale_vec(1,1);
    ang_vel_ratio=OmegaMax/OmegaMin;
    if abs(position_error_norm)>position_epsilon*lin_vel_ratio;
        LinVelMag = Vmax; %go at maximal speed
    elseif abs(position_error_norm)<position_epsilon;
        LinVelMag = 0;
    else
        alpha_translation_t=(position_error_norm - position_epsilon)/...
                            (lin_vel_ratio*position_epsilon - position_epsilon);
        LinVelMag = (Vmax - Vmin)*alpha_translation_t + Vmin;
%         safety check
        if (LinVelMag >Vmax) 
            LinVelMag =Vmax;
        end
    end
    
       
    
    
    if abs(theta_error)>orientation_epsilon*ang_vel_ratio
        alpha_rotation_t=1; %go at maximal speed
    elseif abs(theta_error)<orientation_epsilon,
        alpha_rotation_t=0;
    else
        alpha_rotation_t=theta_error/(ang_vel_ratio*orientation_epsilon);
    end
    
    AngVelMag=alpha_rotation_t*OmegaMax;
    
    % compute desired twist
    x_dot_des = [   LinVelMag*n_unit_vec;
                    AngVelMag*Omega_unit_vec];
    % end
else  %enable=0
    x_dot_des = zeros(6,1);
end
    x_dot_des_disp = x_dot_des;
if DisableOrientation==1
    x_dot_des(4:6) = zeros(3,1);
end
% safety by Long Wang
% check on translation
if (sum(isnan(x_dot_des(1:3)))~=0)
    x_dot_des(1:3,1) = zeros(3,1);
end
if (sum(isnan(x_dot_des(4:6)))~=0)
    x_dot_des(4:6,1) = zeros(3,1);
end

== matlab function Parker 404XR/Magnetic Tracker 125 Hz/process trak1/trakstar_to_pose ==
  data: u input double; sensor output double
function sensor= trak2pose(u)
%#eml
%   Frame definitions:
%   tb: the base frame of trakstar
%   n:  the norm (the X axis of trasmitter)
u = round(u*100)/100;
orig_pos = u(1:3);
n_in_tb = RotationMatrix(u(4),[0;0;1])*RotationMatrix(u(5),[0;1;0])*[1;0;0];
sensor = [orig_pos(:);n_in_tb(:)] ;

== matlab function Trajectory Planner/DaVinci MTM port: 2/UDP_feedback_to_MTM/MSG_Decoding ==
  data: MSG_Type input double; Echo_EN output double
function Echo_EN = Decode(MSG_Type)
%#codegen
% decode the message_type
% MSG_Type def
% bit0 = valid massage or not(enable or not)
% bit1 = time stamping requested or not (if should send back the local time or not)
enable = bitand(uint8(floor(MSG_Type)),2);
Echo_EN= double(enable);

== matlab function Parker 404XR/Magnetic Tracker 125 Hz/process trak2/trakstar_to_pose ==
  data: u input double; sensor output double
function sensor= trak2pose(u)
%#eml
%   Frame definitions:
%   tb: the base frame of trakstar
%   n:  the norm (the X axis of trasmitter)
u = round(u*100)/100;
orig_pos = u(1:3);
n_in_tb = RotationMatrix(u(4),[0;0;1])*RotationMatrix(u(5),[0;1;0])*[1;0;0];
sensor = [orig_pos(:);n_in_tb(:)] ;

== matlab function Parker 404XR/Magnetic Tracker 125 Hz/process trak3/trakstar_to_pose ==
  data: u input double; sensor output double
function sensor= trak2pose(u)
%#eml
%   Frame definitions:
%   tb: the base frame of trakstar
%   n:  the norm (the X axis of trasmitter)
u = round(u*100)/100;
orig_pos = u(1:3);
n_in_tb = RotationMatrix(u(4),[0;0;1])*RotationMatrix(u(5),[0;1;0])*[1;0;0];
sensor = [orig_pos(:);n_in_tb(:)] ;

== matlab function Parker 404XR/Magnetic Tracker 125 Hz/process trak4/trakstar_to_pose ==
  data: u input double; sensor output double
function sensor= trak2pose(u)
%#eml
%   Frame definitions:
%   tb: the base frame of trakstar
%   n:  the norm (the X axis of trasmitter)
u = round(u*100)/100;
orig_pos = u(1:3);
n_in_tb = RotationMatrix(u(4),[0;0;1])*RotationMatrix(u(5),[0;1;0])*[1;0;0];
sensor = [orig_pos(:);n_in_tb(:)] ;
